simulink subsystem "nozzle"  (R2023a)
settings: Solver=VariableStepAuto  StartTime=0.0  StopTime=10.0  RelTol=1e-3
undefined symbols (not defined in the file): rotor, shaftFTP
libraries: fl_lib x2, SimscapeFluids_lib x1, sdl_lib x1
settings Model: Creator=imyrsini  LastModifiedBy=imyrsini

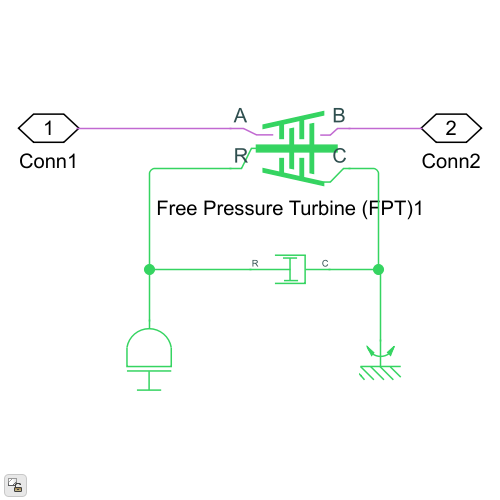
[thumbnail: Simulink's stored preview of the top-level diagram]
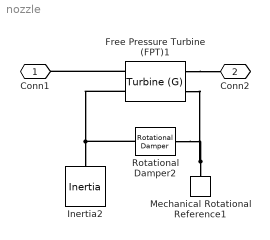
== system nozzle ==
  Free Pressure Turbine (FPT)1 : SimscapeFluids_lib/Gas/Turbomachinery/Turbine (G)  parameterization=fluids.gas.turbomachinery.enum.TurbineParameterization.Analytical  omega_TLU_2=[5000, 6000, 7000, 8000, 9000, 10000, 11000] rpm  variable_nozzle=false  min_nozzle_opening=1e-3  max_nozzle_opening=1  pr_nom=1.2  mdot_nom=turbineFPT.massFlowDesign kg/s  pr_mdot_TLU=[1.251, 1.345, 1.442, 1.521, 1.596, 1.692, 1.849, 1.972, 2.1, 2.173, 2.259, 2.3424]  mdot_TLU=[39.439, 43.01, 45.556, 46.801, 47.792, 48.388, 48.634, 48.67, 48.689, 48.747, 48.825, 48.912] kg/s  pr_mdot_TLU_2=[1.217, 1.285, 1.323, 1.363, 1.402, 1.427, 1.495, 1.545, 1.6, 1.687, 1.747, 1.8074; 1.231, 1.302, 1.356, 1.404, 1.443, 1.473, 1.525, 1.577, 1.635, 1.709, 1.782, 1.845; 1.242, 1.328, 1.388, 1.437, 1.528, 1.617, 1.704, 1.811, 1.915, 1.979, 2.053, 2.1226; 1.244, 1.339, 1.417, 1.465, 1.528, 1.584, 1.692, 1.787, 1.899, 2, 2.075, 2.1492; 1.245, 1.34, 1.425, 1.492, 1.546, 1.684, 1.748, 1.882, 1.987, 2.084, 2.167, 2.2458; 1.251, 1.345, 1.442, 1.521, 1.596, 1.692, 1.849, 1.972, 2.1, 2.173, 2.259, 2.3424; 1.248, 1.348, 1.447, 1.516, 1.581, 1.651, 1.749, 1.839, 1.93, 2.024, 2.154, 2.242]  mdot_TLU_2=[40.403, 44.417, 46.653, 47.966, 48.97, 49.544, 50.001, 50.081, 50.086, 50.095, 50.09, 50.0922; 40.044, 43.754, 46.125, 47.626, 48.513, 49.105, 49.481, 49.58, 49.597, 49.624, 49.638, 49.633; 39.941, 43.795, 46.017, 47.335, 48.795, 49.199, 49.279, 49.27, 49.248, 49.23, 49.255, 49.2428; 39.896, 43.512, 45.914, 47.061, 48.011, 48.558, 48.943, 49.042, 49.069, 49.01, 49.046, 49.0266; 39.524, 42.934, 45.686, 46.743, 47.715, 48.67, 48.777, 48.836, 48.876, 48.836, 48.845, 48.8184; 39.439, 43.01, 45.556, 46.801, 47.792, 48.388, 48.634, 48.67, 48.639, 48.647, 48.625, 48.5912; 39.502, 42.849, 45.336, 46.385, 47.312, 47.877, 48.222, 48.397, 48.459, 48.482, 48.455, 48.414] kg/s  efficiency_constant=turbineFPT.isentropicEfficiency  pr_eta_TLU=[1.252, 1.328, 1.425, 1.544, 1.642, 1.757, 1.873, 2.005, 2.1, 2.204, 2.248, 2.28]  eta_TLU=[.559, .61, .673, .741, .788, .835, .869, .895, .908, .899, .854, .751]  pr_eta_TLU_2=[1.224, 1.246, 1.292, 1.387, 1.457, 1.534, 1.61, 1.686, 1.743, 1.79, 1.871, 1.914; 1.237, 1.25, 1.28, 1.369, 1.459, 1.553, 1.629, 1.716, 1.799, 1.846, 1.927, 1.97; 1.241, 1.255, 1.283, 1.326, 1.401, 1.509, 1.591, 1.704, 1.806, 1.913, 1.994, 2.037; 1.25, 1.265, 1.308, 1.364, 1.456, 1.532, 1.637, 1.739, 1.851, 1.934, 2.042, 2.085; 1.281, 1.314, 1.371, 1.425, 1.498, 1.574, 1.647, 1.749, 1.878, 1.979, 2.091, 2.18; 1.252, 1.328, 1.425, 1.544, 1.642, 1.757, 1.873, 2.005, 2.1, 2.204, 2.248, 2.28; 1.382, 1.43, 1.495, 1.586, 1.688, 1.791, 1.887, 1.99, 2.079, 2.158, 2.249, 2.36]  eta_TLU_2=[.72, .754, .759, .739, .714, .679, .643, .603, .554, .524, .494, .48; .716, .757, .794, .819, .812, .788, .761, .728, .692, .662, .632, .618; .629, .691, .775, .831, .858, .869, .859, .842, .816, .782, .752, .738; .594, .668, .757, .804, .857, .883, .892, .893, .884, .865, .835, .821; .664, .72, .779, .823, .858, .883, .897, .905, .904, .896, .883, .868; .559, .61, .673, .741, .788, .835, .869, .895, .908, .899, .854, .751; .718, .785, .824, .855, .882, .9, .908, .906, .884, .857, .804, .701]  p_reference=turbineFPT.refPressure Pa  T_reference=turbineFPT.refTemperature K  mechanical_efficiency=turbineFPT.mechanicalEff  area_A=coreArea m^2  area_B=coreArea m^2
      settings: InternalSimscapePortConfiguration="{\"Bottom\":[],\"Left\":[{\"id\":\"A\",\"label\":\"A\",\"type\":\"foundation.gas.gas\"},{\"id\":\"R\",\"label\":\"R\",\"type\":\"foundation.mechanical.rotational.rotational\"}],\"Right\":[{\"id\":\"B\",\"label\":\"B\",\"type\":\"foundation.gas.gas\"},{\"id\":\"C\",\"label\":\"C\",\"type\":\"foundation.mechanical.rotational.rotational\"}],\"Top\":[]}"
  Inertia2 : fl_lib/Mechanical/Rotational Elements/Inertia  inertia=shaft.inertia kg*m^2  num_ports=foundation.enum.numPorts2.one  w_specify=on  w_priority=Low  w=shaftFTP.GearRatio*rotor.rpm rpm  w_nominal_specify=off  w_nominal_unit=rad/s  w_nominal_value=1  t_specify=off  t_priority=None  t=0 N*m  t_nominal_specify=off  t_nominal_unit=N*m  t_nominal_value=1
  Mechanical Rotational Reference1 : fl_lib/Mechanical/Rotational Elements/Mechanical Rotational Reference
  Rotational Damper2 : sdl_lib/Couplings & Drives/Springs & Dampers/Rotational Damper  D=1e-3 N*m*s/rad  enable_faults=simscape.enum.onoff.off  b_fault=100 N*m*s/rad  temporal_fault=simscape.enum.onoff.off  fault_time=5 s  shock_fault=simscape.enum.onoff.off  acceleration_limit=100 rad/s^2  shock_limit=1  report_fault=simscape.enum.assert.action.none  thermal_port=simscape.enum.thermaleffects.omit  thermal_mass=50 kJ/K  temperature_specify=off  temperature_priority=High  temperature=300 K  temperature_nominal_specify=off  temperature_nominal_unit=K  temperature_nominal_value=1
  Conn1 : PMIOPort  Side=Left
  Conn2 : PMIOPort  Port=2  Side=Right
  connections:
  Free Pressure Turbine (FPT)1/LConn2 -- Inertia2/LConn1 -- Rotational Damper2/LConn1
  Mechanical Rotational Reference1/LConn1 -- Free Pressure Turbine (FPT)1/RConn2 -- Rotational Damper2/RConn1
  Free Pressure Turbine (FPT)1/LConn1 -- Conn1/RConn1
  Free Pressure Turbine (FPT)1/RConn1 -- Conn2/RConn1
